simulink library "devkit_mpc5744p"  (R2016b)
settings: Solver=VariableStepAuto  StartTime=0.0  StopTime=10.0  RelTol=1e-3
undefined symbols (not defined in the file or in its folder): A15, C12, D17, F12, F13, M14
libraries: devkit_mpc5744p x11, mbd_pnt_ec_toolbox x3, simulink x2
settings Model: Creator=C3038028  LastModifiedBy=C3038028

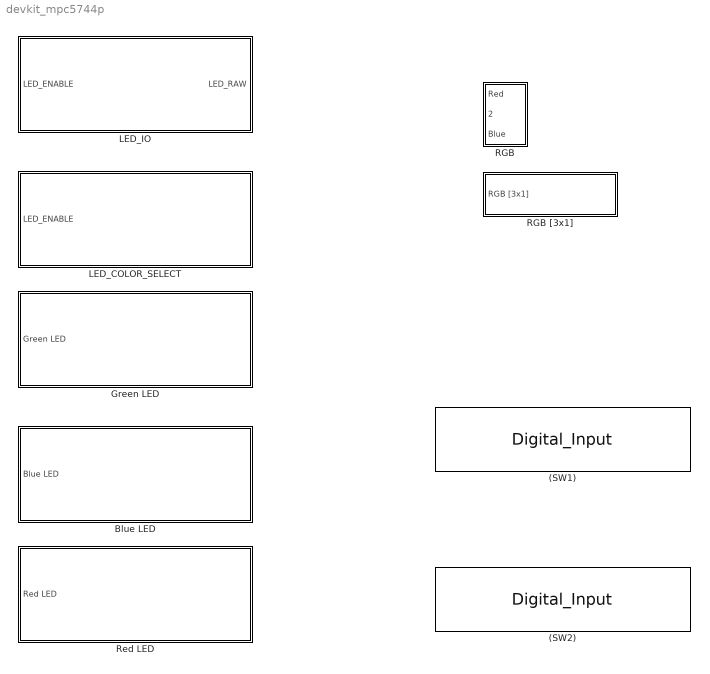
== system devkit_mpc5744p ==
  "(SW1) " : mbd_pnt_ec_toolbox/MPC574xP/Peripheral Interface Blocks/Digital_Input  gpio_outputs="92   : F12 :  [106] : [130] : [D17]"  pinNum=None Selected  pcrNum=92
  (SW2) : mbd_pnt_ec_toolbox/MPC574xP/Peripheral Interface Blocks/Digital_Input  gpio_outputs="93   : F13 :  [112] : [137] : [A15]"  pinNum=None Selected  pcrNum=93
  Blue LED : Subsystem
  Green LED : Subsystem
  LED_COLOR_SELECT : Subsystem  TreatAsAtomicUnit=on  SystemSampleTime=0.1  mask(LED_COLOR_SELECT){led_color=None}
      mask prompts: led_color "LED Color"
      mask help:
      | Select LED Color.
      |
      | Uses: Masks, Parameters, & Callbaks
      mask TypeOptions led_color: None | Red | Green | Blue
      mask Callback led_color: cb_led_select(gcb);
      mask Display: port_label('input', 1, 'LED')
  LED_IO : Subsystem  TreatAsAtomicUnit=on
      settings: RTWFcnNameOpts=Use subsystem name  RTWFileNameOpts=Use subsystem name
  RGB : Subsystem
  RGB [3x1] : Subsystem
  Red LED : Subsystem

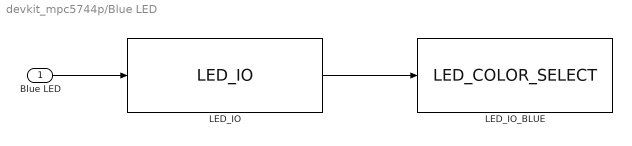
== system devkit_mpc5744p/Blue LED ==
  Blue LED : Inport
  LED_IO : devkit_mpc5744p/LED_IO  SystemSampleTime=-1
  LED_IO_BLUE : devkit_mpc5744p/LED_COLOR_SELECT  led_color=Blue
  wires:
  LED_IO/1 -> LED_IO_BLUE/1
  Blue LED/1 -> LED_IO/1

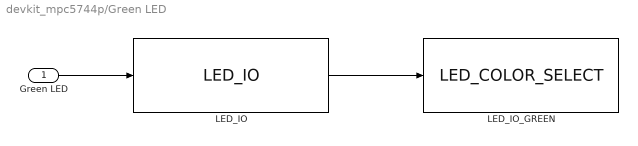
== system devkit_mpc5744p/Green LED ==
  Green LED : Inport
  LED_IO : devkit_mpc5744p/LED_IO  SystemSampleTime=-1
  LED_IO_GREEN : devkit_mpc5744p/LED_COLOR_SELECT  led_color=Green
  wires:
  Green LED/1 -> LED_IO/1
  LED_IO/1 -> LED_IO_GREEN/1

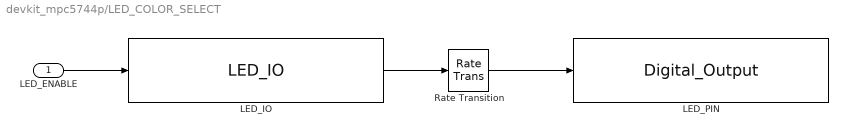
== system devkit_mpc5744p/LED_COLOR_SELECT ==
  LED_ENABLE : Inport
  LED_IO : devkit_mpc5744p/LED_IO  SystemSampleTime=-1
  LED_PIN : mbd_pnt_ec_toolbox/MPC574xP/Peripheral Interface Blocks/Digital_Output  gpio_outputs="44   : C12 :  [82]   : [101] : [M14]"  pinNum=None Selected  pcrNum=44
  Rate Transition : RateTransition
  wires:
  LED_ENABLE/1 -> LED_IO/1
  LED_IO/1 -> Rate Transition/1
  Rate Transition/1 -> LED_PIN/1

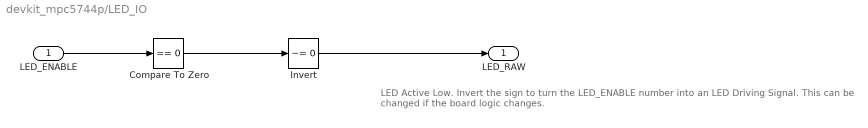
== system devkit_mpc5744p/LED_IO ==
  note: LED Active Low. Invert the sign to turn the LED_ENABLE number into an LED Driving Signal.
      |
      | This can be changed if the board logic changes.
  LED_ENABLE : Inport
  Compare To Zero : simulink/Logic and Bit Operations/Compare To Zero  relop===  OutDataTypeStr=boolean
  Invert : simulink/Logic and Bit Operations/Compare To Zero  relop=~=  OutDataTypeStr=boolean
  LED_RAW : Outport
  wires:
  Invert/1 -> LED_RAW/1
  LED_ENABLE/1 -> Compare To Zero/1
  Compare To Zero/1 -> Invert/1

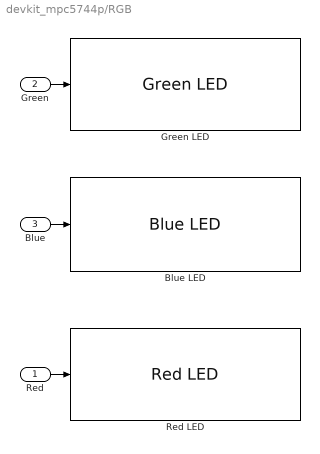
== system devkit_mpc5744p/RGB ==
  Red : Inport
  Green : Inport  Port=2
  Blue : Inport  Port=3
  Blue LED : devkit_mpc5744p/Blue LED
  Green LED : devkit_mpc5744p/Green LED
  Red LED : devkit_mpc5744p/Red LED
  wires:
  Green/1 -> Green LED/1
  Blue/1 -> Blue LED/1
  Red/1 -> Red LED/1

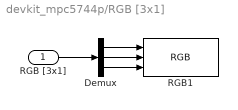
== system devkit_mpc5744p/RGB [3x1] ==
  RGB [3x1] : Inport
  Demux : Demux  Outputs=3
  RGB1 : devkit_mpc5744p/RGB
  wires:
  Demux/3 -> RGB1/3
  Demux/2 -> RGB1/2
  Demux/1 -> RGB1/1
  RGB [3x1]/1 -> Demux/1

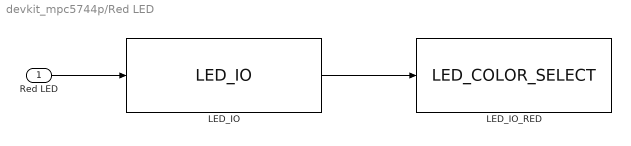
== system devkit_mpc5744p/Red LED ==
  Red LED : Inport
  LED_IO : devkit_mpc5744p/LED_IO  SystemSampleTime=-1
  LED_IO_RED : devkit_mpc5744p/LED_COLOR_SELECT  led_color=Red
  wires:
  Red LED/1 -> LED_IO/1
  LED_IO/1 -> LED_IO_RED/1
